simulink library "util_slosh_lib"  (R2014b)
settings: Solver=ode45  StartTime=0.0  StopTime=10.0  RelTol=1e-3
undefined symbols (not defined in the file or in its folder): sim_time_step_size, SloshData
undefined symbols (not defined in the file): mpl_htp_center_tank1, mpl_htp_mass_fillfrac_100, mpl_htp_tank_radius, slh_damping_enable, slh_forces_enable, slh_htp_phi_2dot_limit, slh_IC_settle_time, slh_moments_enable
libraries: util_common_lib x6, simulink_extras x2, util_quat_lib x2
settings Model: Creator=Mark Agbayani  LastModifiedBy=Mark Agbayani

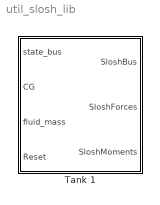
== system util_slosh_lib ==
  Tank 1 : Subsystem  mask{forces_enable=slh_forces_enable, moments_enable=slh_moments_enable, damping_enable=slh_damping_enable, phi_2dot_limit=slh_htp_phi_2dot_limit, mass_fillfrac_100=mpl_htp_mass_fillfrac_100, tank_radius=mpl_htp_tank_radius, tank_center=mpl_htp_center_tank1, IC_settle_time=slh_IC_settle_time}
      mask prompts: forces_enable "Slosh Forces Enable/Disable"; moments_enable "Slosh Moments Enable/Disable"; damping_enable "Fluid Damping Enable/Disable"; phi_2dot_limit "Fluid Rotational Acceleration Limit, rad/sec"; mass_fillfrac_100 "Fluid Mass at 100 Percent Fill, kg"; tank_radius "Tank Radius,  m"; tank_center "Tank Center Location [x y z],  m"; IC_settle_time "Initial Condition Settling Time, sec"
      mask help:
      | Slosh is modeled using a spherical pendulum mechanical system.
      |
      | This block models the first slosh mode for a single tank of fluid.
      |
      | The outputs of this model are the forces and moments acting
      | at the pendulum hinge.
      mask Display:
      | color('blue')
      | text(0.05,0.02,'MoonEx',...
      |  	'HorizontalAlignment','Left',...
      | 	'VerticalAlignment','bottom')

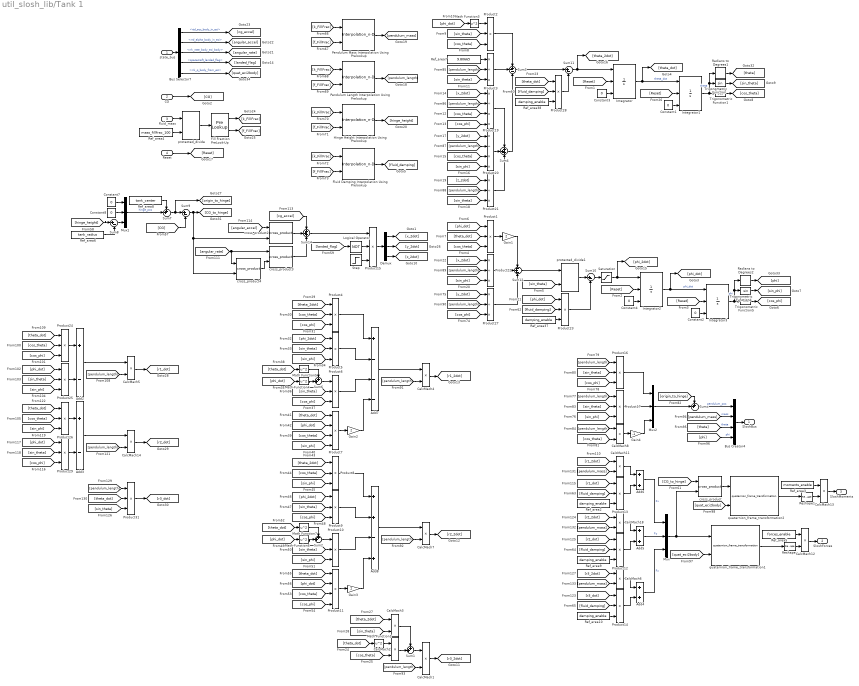
== system util_slosh_lib/Tank 1 ==
  state_bus : Inport
  CG : Inport  Port=2
  fluid_mass : Inport  Port=3
  Reset : Inport  Port=4
  Add2 : Sum  Inputs=+-
  Add3 : Sum  Inputs=+-
  Add4 : Sum
  Add5 : Sum
  Add6 : Sum
  Add7 : Sum  Inputs=+---
  Add8 : Sum  Inputs=++-+
  Bus Creator4 : BusCreator
  Bus Selector7 : BusSelector  OutputSignals=rtd_acc_body_in_eci,rrd_alpha_body_in_eci,rrk_rate_body_eci_body,spacecraft_landed_flag,rrk_q_body_from_eci
  CalcMach{1..8,11..14,18} (13 alike) : Product  SaturateOnIntegerOverflow=on  OutDataTypeStr=Inherit: Same as first input
  Constant{1..4} (4 alike) : Constant  Value=0  VectorParams1D=off
  Constant7 : Constant  Value=0
  Constant8 : Constant  Value=0
  Demux : Demux  Outputs=3
  Fill Fraction PreLook-Up : PreLookup  BreakpointsData=SloshData.fill_fraction  BeginIndexSearchUsingPreviousIndexResult=on
  Fluid Damping Interpolation Using Prelookup : Interpolation_n-D  NumberOfTableDimensions=1  Table=SloshData.fluid_damping  ExtrapMethod=Clip  InternalRulePriority=Speed
      settings: InputPortMap=u0,u1
  Gain1 : Gain  Gain=2
  Gain2 : Gain  Gain=2
  Gain3 : Gain  Gain=2
  Gain4 : Gain  Gain=-1
  Hinge Height Interpolation Using Prelookup : Interpolation_n-D  NumberOfTableDimensions=1  Table=SloshData.hinge_height  ExtrapMethod=Clip  InternalRulePriority=Speed
      settings: InputPortMap=u0,u1
  Integrator{,1..3} (4 alike) : Integrator  ExternalReset=rising  InitialConditionSource=external
  Logical Operator : Logic  Operator=NOT  AllPortsSameDT=off  OutDataTypeStr=boolean
  Math Function{1,3..7} (6 alike) : Math  Operator=square  SaturateOnIntegerOverflow=on
  Mux : Mux  Inputs=3
  Mux1 : Mux  Inputs=3
  Mux2 : Mux  Inputs=3
  Pendulum Length Interpolation Using Prelookup : Interpolation_n-D  NumberOfTableDimensions=1  Table=SloshData.pendulum_length  ExtrapMethod=Clip  InternalRulePriority=Speed
      settings: InputPortMap=u0,u1
  Pendulum Mass Interpolation Using Prelookup : Interpolation_n-D  NumberOfTableDimensions=1  Table=SloshData.pendulum_mass  ExtrapMethod=Clip  InternalRulePriority=Speed
      settings: InputPortMap=u0,u1
  Product{1..2,4..6,8..10,12..17,23..26,28..29,31} (21 alike) : Product  Inputs=***  RndMeth=Zero
  Product11 : Product  Inputs=****  RndMeth=Zero
  Product19 : Product  Inputs=*/**  RndMeth=Zero
  Product20 : Product  Inputs=*/**  RndMeth=Zero
  Product{3,21..22,27} (4 alike) : Product  Inputs=*/*  RndMeth=Zero
  Product7 : Product  Inputs=****  RndMeth=Zero
  Radians to Degrees1 : simulink_extras/Transformations/Radians to Degrees
  Radians to Degrees2 : simulink_extras/Transformations/Radians to Degrees
  Ref_area{2,9..10,37..38} (5 alike) : Constant  Value=damping_enable
  Ref_area3 : Constant  Value=moments_enable
  Ref_area4 : Constant  Value=mass_fillfrac_100
  Ref_area5 : Constant  Value=forces_enable
  Ref_area6 : Constant  Value=tank_radius
  Ref_area7 : Constant  Value=9.80665
  Ref_area8 : Constant  Value=tank_center
  Reshape : Reshape
  Reshape1 : Reshape
  Saturation : Saturate  UpperLimit=phi_2dot_limit  LowerLimit=-phi_2dot_limit
  Step : Step  Time=IC_settle_time  SampleTime=sim_time_step_size
  Sum{1..2,5..7} (5 alike) : Sum  Inputs=++|
  Sum{8..11} (4 alike) : Sum  Inputs=|+-
  Sum12 : Sum  Inputs=-+-
  Sum14 : Sum  Inputs=+++
  Sum3 : Sum  Inputs=+--
  Sum4 : Sum  Inputs=+++
  Trigonometric Function : Trigonometry
  Trigonometric Function1 : Trigonometry  Operator=cos
  Trigonometric Function4 : Trigonometry
  Trigonometric Function5 : Trigonometry  Operator=cos
  cross_product{,2..4} (4 alike) : util_common_lib/cross_product  SystemSampleTime=-1
  protected_divide : util_common_lib/protected_divide  fault_value=0  tolerance=eps
  protected_divide1 : util_common_lib/protected_divide  fault_value=0  tolerance=eps
  quaternion_frame_transformation1 : util_quat_lib/quaternion_frame_transformation  SystemSampleTime=-1
  quaternion_frame_transformation2 : util_quat_lib/quaternion_frame_transformation  SystemSampleTime=-1
  SloshBus : Outport
  SloshForces : Outport  Port=2
  SloshMoments : Outport  Port=3
  wires:
  CalcMach13/1 -> SloshMoments/1
  CalcMach12/1 -> SloshForces/1
  quaternion_frame_transformation1/1 -> Reshape/1
  Reshape/1 -> CalcMach12/2
  Ref_area5/1 -> CalcMach12/1
  quaternion_frame_transformation2/1 -> Reshape1/1
  Ref_area3/1 -> CalcMach13/1
  Reshape1/1 -> CalcMach13/2
  Sum5/1 -> Bus Creator4/1  "pendulum_pos"
  [quat_eci2body] -> quaternion_frame_transformation2/2
  [quat_eci2body] -> quaternion_frame_transformation1/2
  Bus Selector7/5 -> [quat_eci2body]  "<rrk_q_body_from_eci>"
  [phi] -> Bus Creator4/4  "phi"
  [theta] -> Bus Creator4/3  "theta"
  Radians to Degrees2/1 -> [phi]
  Radians to Degrees1/1 -> [theta]
  Sum7/1 -> Sum9/1, [origin_to_hinge]
  Bus Creator4/1 -> SloshBus/1
  [pendulum_mass] -> Bus Creator4/2  "mass"
  [origin_to_hinge] -> Sum5/1
  Gain4/1 -> Mux2/3
  [cos_theta] -> CalcMach8/2
  [pendulum_length] -> Product17/1
  Mux2/1 -> Sum5/2
  CalcMach8/1 -> Gain4/1
  Product16/1 -> Mux2/1
  Product17/1 -> Mux2/2
  [cos_phi] -> Product16/3
  [pendulum_length] -> Product16/1
  [sin_theta] -> Product16/2
  [sin_theta] -> Product17/2
  [sin_phi] -> Product17/3
  [pendulum_length] -> CalcMach8/1
  Logical Operator/1 -> Product15/2
  Bus Selector7/4 -> [landed_flag]  "<spacecraft_landed_flag>"
  Sum14/1 -> Product15/1
  [landed_flag] -> Logical Operator/1
  Step/1 -> Product15/3
  Product15/1 -> Demux/1
  Sum9/1 -> cross_product2/2, cross_product4/2, [CG_to_hinge]
  Demux/3 -> [z_2dot]
  Demux/2 -> [y_2dot]
  Demux/1 -> [x_2dot]
  [cg_accel] -> Sum14/1
  cross_product3/1 -> Sum14/3
  cross_product2/1 -> Sum14/2
  [angular_accel] -> cross_product2/1
  [angular_rate] -> cross_product4/1, cross_product3/1
  cross_product4/1 -> cross_product3/2
  CG/1 -> [CG]
  Reset/1 -> [Reset]
  Hinge Height Interpolation Using Prelookup/1 -> [hinge_height]
  Pendulum Length Interpolation Using Prelookup/1 -> [pendulum_length]
  Constant3/1 -> Integrator/3
  Constant1/1 -> Integrator1/3
  Integrator/1 -> Integrator1/1, [theta_dot]  "theta_dot"
  [Reset] -> Integrator1/2
  [Reset] -> Integrator/2
  Constant4/1 -> Integrator2/3
  Constant2/1 -> Integrator3/3
  Integrator2/1 -> Integrator3/1, [phi_dot]  "phi_dot"
  [Reset] -> Integrator3/2
  [Reset] -> Integrator2/2
  Integrator3/1 -> Trigonometric Function4/1, Radians to Degrees2/1, Trigonometric Function5/1  "phi"
  Saturation/1 -> Integrator2/1, [phi_2dot]
  Sum11/1 -> Integrator/1, [theta_2dot]
  Math Function3/1 -> Product2/1
  [phi_dot] -> Math Function3/1
  Product2/1 -> Sum3/1
  Product3/1 -> Sum3/2
  CalcMach1/1 -> [r3_2dot]
  Sum1/1 -> CalcMach1/1
  CalcMach2/1 -> Sum1/2
  Math Function1/1 -> CalcMach2/1
  [theta_dot] -> Math Function1/1
  [cos_theta] -> CalcMach2/2
  [theta_2dot] -> CalcMach3/1
  [sin_theta] -> CalcMach3/2
  CalcMach3/1 -> Sum1/1
  CalcMach4/1 -> [r1_2dot]
  Add7/1 -> CalcMach4/1
  [theta_2dot] -> Product4/1
  [cos_theta] -> Product4/2
  [cos_phi] -> Product4/3
  [phi_2dot] -> Product5/1
  [sin_theta] -> Product5/2
  [sin_phi] -> Product5/3
  [sin_theta] -> Product6/2
  [cos_phi] -> Product6/3
  [phi_dot] -> Math Function4/1
  Sum6/1 -> Product6/1
  Math Function4/1 -> Sum6/2
  [theta_dot] -> Math Function5/1
  Math Function5/1 -> Sum6/1
  [sin_phi] -> Product7/4
  Product4/1 -> Add7/1
  Gain2/1 -> Add7/4
  Product6/1 -> Add7/3
  Product5/1 -> Add7/2
  CalcMach7/1 -> [r2_2dot]
  [theta_2dot] -> Product8/1
  [cos_theta] -> Product8/2
  [sin_phi] -> Product8/3
  [phi_2dot] -> Product9/1
  [sin_theta] -> Product9/2
  [cos_phi] -> Product9/3
  [sin_theta] -> Product10/2
  [sin_phi] -> Product10/3
  [phi_dot] -> Math Function6/1
  Sum2/1 -> Product10/1
  Math Function6/1 -> Sum2/2
  [theta_dot] -> Math Function7/1
  Math Function7/1 -> Sum2/1
  Product8/1 -> Add8/1
  Gain3/1 -> Add8/4
  Product10/1 -> Add8/3
  Product9/1 -> Add8/2
  Add6/1 -> Mux/1  "Fx"
  Add5/1 -> Mux/2  "Fy"
  Add4/1 -> Mux/3  "Fz"
  fluid_mass/1 -> protected_divide/1
  Product19/1 -> Sum4/1
  [x_2dot] -> Product19/1
  Product20/1 -> Sum4/2
  Product21/1 -> Sum4/3
  [cos_theta] -> Product7/3
  [theta_dot] -> Product7/1
  [phi_dot] -> Product7/2
  Product7/1 -> Gain2/1
  [cos_phi] -> Product11/4
  [cos_theta] -> Product11/3
  [theta_dot] -> Product11/1
  [phi_dot] -> Product11/2
  [y_2dot] -> Product27/1
  [x_2dot] -> Product22/1
  [cos_theta] -> Product1/3
  [phi_dot] -> Product1/1
  [theta_dot] -> Product1/2
  [pendulum_length] -> Product22/2
  [sin_phi] -> Product22/3
  [pendulum_length] -> Product27/2
  [cos_phi] -> Product27/3
  Product11/1 -> Gain3/1
  Add8/1 -> CalcMach7/1
  Product1/1 -> Gain1/1
  [pendulum_length] -> Product21/2
  [sin_theta] -> Product21/3
  [pendulum_length] -> Product20/2
  [cos_theta] -> Product20/3
  [sin_phi] -> Product20/4
  [pendulum_length] -> Product19/2
  [cos_theta] -> Product19/3
  [cos_phi] -> Product19/4
  [z_2dot] -> Product21/1
  [y_2dot] -> Product20/1
  Ref_area7/1 -> Product3/1
  [pendulum_length] -> Product3/2
  [sin_theta] -> Product3/3
  [sin_theta] -> Product2/2
  [cos_theta] -> Product2/3
  [sin_theta] -> protected_divide1/2
  [phi_dot] -> Product23/1
  [fluid_damping] -> Product23/2
  Product23/1 -> Sum10/2
  [theta_dot] -> Product28/1
  [fluid_damping] -> Product28/2
  Product28/1 -> Sum11/2
  Sum3/1 -> Sum11/1
  Sum4/1 -> Sum3/3
  Gain1/1 -> Sum12/1
  Product27/1 -> Sum12/3
  Product22/1 -> Sum12/2
  Integrator1/1 -> Trigonometric Function/1, Radians to Degrees1/1, Trigonometric Function1/1  "theta"
  Ref_area37/1 -> Product23/3
  Ref_area38/1 -> Product28/3
  [pendulum_length] -> CalcMach1/2
  [pendulum_length] -> CalcMach7/2
  [pendulum_length] -> CalcMach4/2
  Sum10/1 -> Saturation/1
  Pendulum Mass Interpolation Using Prelookup/1 -> [pendulum_mass]
  Sum12/1 -> protected_divide1/1
  protected_divide1/1 -> Sum10/1
  Mux/1 -> cross_product/2, quaternion_frame_transformation1/1
  cross_product/1 -> quaternion_frame_transformation2/1
  Ref_area4/1 -> protected_divide/2
  protected_divide/1 -> Fill Fraction PreLook-Up/1
  state_bus/1 -> Bus Selector7/1
  Bus Selector7/3 -> [angular_rate]  "<rrk_rate_body_eci_body>"
  Bus Selector7/2 -> [angular_accel]  "<rrd_alpha_body_in_eci>"
  Bus Selector7/1 -> [cg_accel]  "<rtd_acc_body_in_eci>"
  Add2/1 -> CalcMach5/1
  [pendulum_length] -> CalcMach5/2
  [theta_dot] -> Product24/1
  [cos_theta] -> Product24/2
  [cos_phi] -> Product24/3
  Product24/1 -> Add2/1
  [phi_dot] -> Product25/1
  [sin_theta] -> Product25/2
  [sin_phi] -> Product25/3
  Product25/1 -> Add2/2
  Add3/1 -> CalcMach14/1
  [pendulum_length] -> CalcMach14/2
  [theta_dot] -> Product26/1
  [cos_theta] -> Product26/2
  [cos_phi] -> Product29/3
  Product26/1 -> Add3/1
  [phi_dot] -> Product29/1
  [sin_theta] -> Product29/2
  [sin_phi] -> Product26/3
  Product29/1 -> Add3/2
  [pendulum_length] -> Product31/1
  [theta_dot] -> Product31/2
  [sin_theta] -> Product31/3
  CalcMach11/1 -> Add6/1
  [pendulum_mass] -> CalcMach11/2
  [r1_2dot] -> CalcMach11/1
  CalcMach18/1 -> Add5/1
  [pendulum_mass] -> CalcMach18/2
  [r2_2dot] -> CalcMach18/1
  [pendulum_mass] -> CalcMach6/2
  [r3_2dot] -> CalcMach6/1
  CalcMach6/1 -> Add4/1
  [fluid_damping] -> Product14/2
  [r3_dot] -> Product14/1
  Product14/1 -> Add4/2
  [fluid_damping] -> Product12/2
  [r2_dot] -> Product12/1
  Product12/1 -> Add5/2
  [fluid_damping] -> Product13/2
  [r1_dot] -> Product13/1
  Product13/1 -> Add6/2
  Trigonometric Function/1 -> [sin_theta]
  Trigonometric Function1/1 -> [cos_theta]
  Trigonometric Function4/1 -> [sin_phi]
  Trigonometric Function5/1 -> [cos_phi]
  CalcMach5/1 -> [r1_dot]
  CalcMach14/1 -> [r2_dot]
  Product31/1 -> [r3_dot]
  [CG] -> Sum9/2
  Mux1/1 -> Sum7/2  "hinge_pos"
  Ref_area8/1 -> Sum7/1
  Sum8/1 -> Mux1/3
  Constant7/1 -> Mux1/1
  Constant8/1 -> Mux1/2
  Ref_area6/1 -> Sum8/2
  [hinge_height] -> Sum8/1
  [CG_to_hinge] -> cross_product/1
  Fluid Damping Interpolation Using Prelookup/1 -> [fluid_damping]
  Ref_area2/1 -> Product13/3
  Ref_area9/1 -> Product12/3
  Ref_area10/1 -> Product14/3
  Fill Fraction PreLook-Up/1 -> [k_FillFrac]
  Fill Fraction PreLook-Up/2 -> [f_FillFrac]
  [k_FillFrac] -> Pendulum Mass Interpolation Using Prelookup/1
  [f_FillFrac] -> Pendulum Mass Interpolation Using Prelookup/2
  [k_FillFrac] -> Pendulum Length Interpolation Using Prelookup/1
  [f_FillFrac] -> Pendulum Length Interpolation Using Prelookup/2
  [k_FillFrac] -> Hinge Height Interpolation Using Prelookup/1
  [f_FillFrac] -> Hinge Height Interpolation Using Prelookup/2
  [k_FillFrac] -> Fluid Damping Interpolation Using Prelookup/1
  [f_FillFrac] -> Fluid Damping Interpolation Using Prelookup/2
